simulink model "Lqr_simulink"  (R2019a)
settings: Solver=VariableStepAuto  StartTime=0.0  StopTime=15  RelTol=1e-3
values from neighbouring files (symbols this model uses):
  A = [0, 0, 1, 0 ... (first row only)    [Base_proyecto.m]    (also in lqr_proyecto.m)
  B = [0 ... (first row only)    [Base_proyecto.m]    (also in lqr_proyecto.m)
  K = lqr(A,B,Q,R)    [Base_proyecto.m]    (also in lqr_proyecto.m)
libraries: simulink x1
settings Model: Creator=WALTER  LastModifiedBy=WALTER

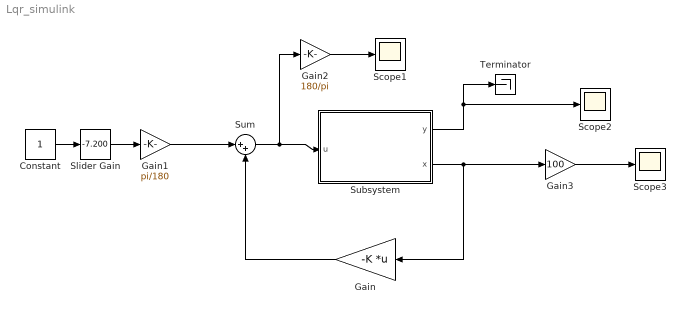
== system Lqr_simulink ==
  Constant : Constant
  Gain : Gain  Gain=-K  Multiplication=Matrix(K*u)
  Gain1 : Gain  Gain=pi/180
  Gain2 : Gain  Gain=180/pi
  Gain3 : Gain  Gain=100
  Scope1 : Scope
  Scope2 : Scope
  Scope3 : Scope
  Slider Gain : simulink/Math Operations/Slider Gain  gain=-7.200  low=-20  high=20
  Subsystem : Subsystem
  Sum : Sum  Inputs=|++
  Terminator : Terminator
  wires:
  Gain/1 -> Sum/2
  Sum/1 -> Gain2/1, Subsystem/1(u)
  Slider Gain/1 -> Gain1/1
  Constant/1 -> Slider Gain/1
  Gain1/1 -> Sum/1
  Subsystem/1(y) -> Scope2/1, Terminator/1
  Gain2/1 -> Scope1/1
  Subsystem/2(x) -> Gain3/1, Gain/1
  Gain3/1 -> Scope3/1

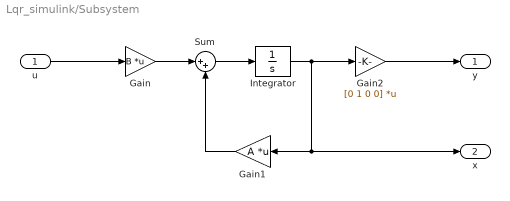
== system Lqr_simulink/Subsystem ==
  u : Inport
  Gain : Gain  Gain=B  Multiplication=Matrix(K*u)
  Gain1 : Gain  Gain=A  Multiplication=Matrix(K*u) (u vector)
  Gain2 : Gain  Gain=[0 1 0 0]  Multiplication=Matrix(K*u) (u vector)
  Integrator : Integrator
  Sum : Sum  Inputs=|++
  y : Outport
  x : Outport  Port=2
  wires:
  Gain1/1 -> Sum/2
  Gain/1 -> Sum/1
  Integrator/1 -> x/1, Gain1/1, Gain2/1
  Gain2/1 -> y/1
  Sum/1 -> Integrator/1
  u/1 -> Gain/1
